simulink model "Backups"  (R2020b)
settings: Solver=VariableStepAuto  StartTime=0.0  StopTime=10.0  RelTol=1e-3
undefined symbols (not defined in the file): O, P_Blowdown, P_Needleboi
libraries: pid_lib x3, simulink x1, dspfdesign x1
(part 1 of 2)
settings Model: Creator=parthmahendru  LastModifiedBy=parthmahendru

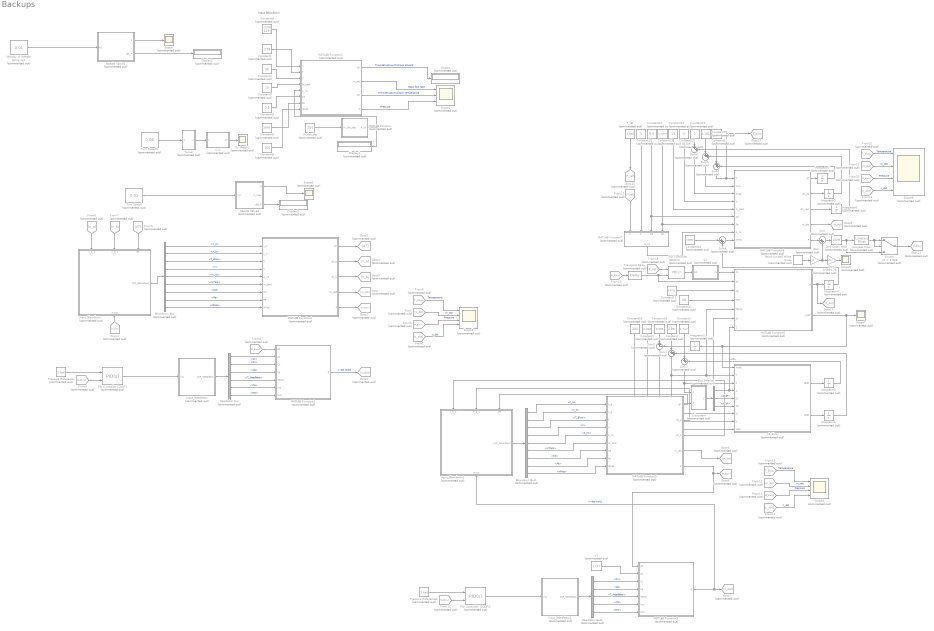
== system Backups ==
  note: Input Blowdown
  Band-Limited White Noise : simulink/Sources/Band-Limited White Noise  Commented=on  Cov=100000  Ts=0.001  seed=[23341]
  Blowdown Bus : BusSelector  Commented=on  OutputSignals=n_a,n_b,T_Blow,V,A_inj,mTank,Cd,Pe,nPres
  Blowdown Bus1 : BusSelector  Commented=on  OutputSignals=n_a,n_b,T_Blow,V,A_inj,mTank,Cd,Pe,nPres
  Bus Selector : BusSelector  Commented=on  OutputSignals=Z,dZdT,dZdP
  Constant : Constant  Commented=on  Value=298
  Constant1 : Constant  Commented=on  Value=278
  Constant10 : Constant  Commented=on
  Constant11 : Constant  Commented=on  Value=0.9723
  Constant12 : Constant  Commented=on  Value=28
  Constant13 : Constant  Commented=on  Value=10
  Constant14 : Constant  Commented=on  Value=0.0032
  Constant15 : Constant  Commented=on  Value=2.413e6  VectorParams1D=off
  Constant16 : Constant  Commented=on  Value=200
  Constant17 : Constant  Commented=on  Value=0.5
  Constant18 : Constant  Commented=on  Value=0.555
  Constant19 : Constant  Commented=on  Value=0.181
  Constant2 : Constant  Commented=on  Value=1.7e7
  Constant20 : Constant  Commented=on  Value=0.01108
  Constant21 : Constant  Commented=on  Value=0
  Constant22 : Constant  Commented=on  Value=278
  Constant3 : Constant  Commented=on  Value=30
  Constant4 : Constant  Commented=on  Value=[250 125]
  Constant5 : Constant  Commented=on  Value=10
  Constant6 : Constant  Commented=on  Value=20000
  Constant7 : Constant  Commented=on  Value=0.003
  Constant8 : Constant  Commented=on  Value=100
  Constant9 : Constant  Commented=on  Value=0.5
  Cv : Subsystem  Commented=on
  Cv Graph2 : Scope  Commented=on
  Cv1 : MATLAB Function  Commented=on  TreatAsAtomicUnit=on
  Display{,1..3} (4 alike) : Display  Commented=on
  From : From  Commented=on  GotoTag=m_dot
  From{1..2,11,16} (4 alike) : From  Commented=on  GotoTag=n_dot
  From10 : From  Commented=on  GotoTag=m_dot
  From{3..5,12..13,19..20} (7 alike) : From  Commented=on  GotoTag=P_Blow
  From14 : From  Commented=on  GotoTag=T_blow  TagVisibility=global
  From15 : From  Commented=on  GotoTag=m_dot
  From17 : From  Commented=on  GotoTag=P_ref
  From18 : From  Commented=on  GotoTag=P_ref
  From21 : From  Commented=on  GotoTag=T_blow  TagVisibility=global
  From6 : From  Commented=on  GotoTag=T_blow  TagVisibility=global
  From7 : From  Commented=on  GotoTag=n_b
  From8 : From  Commented=on  GotoTag=n_a
  From9 : From  Commented=on  GotoTag=dT
  Gain : Gain  Commented=on  Gain=4
  Gain1 : Gain  Commented=on  Gain=1/6894.76
  Goto : Goto  Commented=on  GotoTag=m_dot
  Goto1 : Goto  Commented=on  GotoTag=n_dot
  Goto10 : Goto  Commented=on  GotoTag=n_dot
  Goto11 : Goto  Commented=on  GotoTag=P_Blow
  Goto12 : Goto  Commented=on  GotoTag=T_blow  TagVisibility=global
  Goto13 : Goto  Commented=on  GotoTag=P_ref
  Goto2 : Goto  Commented=on  GotoTag=P_Blow
  Goto3 : Goto  Commented=on  GotoTag=n_b
  Goto4 : Goto  Commented=on  GotoTag=n_a
  Goto5 : Goto  Commented=on  GotoTag=dT
  Goto6 : Goto  Commented=on  GotoTag=m_dot
  Goto7 : Goto  Commented=on  GotoTag=n_dot
  Goto8 : Goto  Commented=on  GotoTag=P_Blow
  Goto9 : Goto  Commented=on  GotoTag=m_dot
  Input_Blowdown : Subsystem  Commented=on
      settings: PortSchema="{\"entries\":[{\"content\":{\"sides\":[{\"content\":{\"connectorIds\":[]},\"type\":\"ConnectorPlacement.EquallySpacedRectSide\",\"uuid\":\"6a11c464-4778-4366-9c52-25a6635196e9\"},{\"content\":{\"connectorIds\":[\"Out1\"],\"side\":\"RIGHT\"},\"type\":\"ConnectorPlacement.EquallySpacedRectSide\",\"uuid\":\"71180da6-79ed-43c5-a069-02da8079ba8e\"},{\"content\":{\"connectorIds\":[\"In1\",\"In2\",\"In3\"],\"side\":\"TOP\"},\"type\":\"ConnectorPlacement.EquallySpacedRectSide\",\"uuid\":\"0f5fbdd2-8e41-48bf-ac62-c31d274b4c94\"},{\"content\":{\"connectorIds\":[\"In4\"],\"side\":\"BOTTOM\"},\"type\":\"ConnectorPlacement.EquallySpacedRectSide\",\"uuid\":\"7608bf70-ac84-4a07-a3b2-996f245fbd8b\"}]},\"type\":\"ConnectorPlacement.EquallySpacedConnector\",\"uuid\":\"0ffd5217-2610-43b0-91a4-99377aa3c0d2\"}],\"packageUris\":[\"http://schema.mathworks.com/mf0/Connector/19700101\"],\"version\":\"1.0\"}"
  Input_Blowdown1 : Subsystem  Commented=on
      settings: PortSchema="{\"entries\":[{\"content\":{\"sides\":[{\"content\":{\"connectorIds\":[]},\"type\":\"ConnectorPlacement.EquallySpacedRectSide\",\"uuid\":\"6a11c464-4778-4366-9c52-25a6635196e9\"},{\"content\":{\"connectorIds\":[\"Out1\"],\"side\":\"RIGHT\"},\"type\":\"ConnectorPlacement.EquallySpacedRectSide\",\"uuid\":\"71180da6-79ed-43c5-a069-02da8079ba8e\"},{\"content\":{\"connectorIds\":[\"In1\",\"In2\",\"In3\"],\"side\":\"TOP\"},\"type\":\"ConnectorPlacement.EquallySpacedRectSide\",\"uuid\":\"0f5fbdd2-8e41-48bf-ac62-c31d274b4c94\"},{\"content\":{\"connectorIds\":[\"In4\"],\"side\":\"BOTTOM\"},\"type\":\"ConnectorPlacement.EquallySpacedRectSide\",\"uuid\":\"7608bf70-ac84-4a07-a3b2-996f245fbd8b\"}]},\"type\":\"ConnectorPlacement.EquallySpacedConnector\",\"uuid\":\"0ffd5217-2610-43b0-91a4-99377aa3c0d2\"}],\"packageUris\":[\"http://schema.mathworks.com/mf0/Connector/19700101\"],\"version\":\"1.0\"}"
  Input_Needleboi : Subsystem  Commented=on
  Input_Needleboi1 : Subsystem  Commented=on
  Integrator{1..7} (7 alike) : Integrator  Commented=on
  Lowpass Filter : dspfdesign/Lowpass Filter  Commented=on  FilterType=FIR  DesignForMinimumOrder=off  FilterOrder=10  PassbandFrequency=700  StopbandFrequency=3000  PassbandRipple=0.1  StopbandAttenuation=80  InheritSampleRate=off  SampleRate=44100  SimulateUsing=Interpreted execution  roundingMode=Nearest  coeffsDataTypeStr=fixdt(1,16)
  MATLAB Function : MATLAB Function  Commented=on  TreatAsAtomicUnit=on
  MATLAB Function1 : MATLAB Function  Commented=on  TreatAsAtomicUnit=on
  MATLAB Function2 : MATLAB Function  Commented=on  TreatAsAtomicUnit=on
  MATLAB Function3 : MATLAB Function  Commented=on  TreatAsAtomicUnit=on
  MATLAB Function4 : MATLAB Function  Commented=on  TreatAsAtomicUnit=on
  MATLAB Function5 : MATLAB Function  Commented=on  TreatAsAtomicUnit=on
  MATLAB Function6 : MATLAB Function  Commented=on  TreatAsAtomicUnit=on
  MATLAB Function7 : MATLAB Function  Commented=on  TreatAsAtomicUnit=on
  MATLAB Function8 : MATLAB Function  Commented=on  TreatAsAtomicUnit=on
  Needle Valve1 : Subsystem  Commented=on
  Needle Valve3 : Subsystem  Commented=on
  Needleboi Bus : BusSelector  Commented=on  OutputSignals=p1,Cv,sg,T_Needleboi,rho,MW
  Needleboi Bus1 : BusSelector  Commented=on  OutputSignals=Cv,sg,T_Needleboi,rho,MW
  PID Controller (2DOF) : pid_lib/PID Controller (2DOF)  Commented=on  Controller=PID  Form=Parallel  TimeDomain=Continuous-time  UseExternalTs=off  SampleTime=-1  IntegratorMethod=Forward Euler  FilterMethod=Forward Euler  ControllerParametersSource=internal  P=4.2846829311871e-09  I=2.39281882332403e-13  D=1.70470224737219e-05  UseFilter=on  N=1.09398371936337  b=1  c=1  TunerSelectOption=Transfer Function Based (PID Tuner App)  InitialConditionSource=internal  InitialConditionForIntegrator=0  InitialConditionForFilter=0  DifferentiatorICPrevScaledInput=0  ExternalReset=none  TrackingMode=off  Kt=1  LimitOutput=on  SatLimitsSource=internal  UpperSaturationLimit=5  LowerSaturationLimit=0  LinearizeAsGain=on  AntiWindupMode=none  Kb=1  POutMin=[]  POutMax=[]  IOutMin=[]  IOutMax=[]  DOutMin=[]  DOutMax=[]  NOutMin=[]  NOutMax=[]  bOutMin=[]  bOutMax=[]  cOutMin=[]  cOutMax=[]  SumOutMin=[]  SumOutMax=[]  SaturationOutMin=[]  SaturationOutMax=[]  PParamMin=[]  PParamMax=[]  IParamMin=[]  IParamMax=[]  DParamMin=[]  DParamMax=[]  NParamMin=[]  NParamMax=[]  bParamMin=[]  bParamMax=[]  cParamMin=[]  cParamMax=[]  KbParamMin=[]  KbParamMax=[]  KtParamMin=[]  KtParamMax=[]  KbOutMin=[]  KbOutMax=[]  KtOutMin=[]  KtOutMax=[]  IntegratorOutMin=[]  IntegratorOutMax=[]  FilterOutMin=[]  FilterOutMax=[]  SumI1OutMin=[]  SumI1OutMax=[]  SumI2OutMin=[]  SumI2OutMax=[]  SumI3OutMin=[]  SumI3OutMax=[]  SumI4OutMin=[]  SumI4OutMax=[]  SumDOutMin=[]  SumDOutMax=[]  Sum1OutMin=[]  Sum1OutMax=[]  Sum2OutMin=[]  Sum2OutMax=[]  Sum3OutMin=[]  Sum3OutMax=[]  DifferentiatorOutMin=[]  DifferentiatorOutMax=[]  FilterDiffOutCoefMin=[]  FilterDiffOutCoefMax=[]  ReciprocalOutMin=[]  ReciprocalOutMax=[]  SumDenOutMin=[]  SumDenOutMax=[]  SumNumOutMin=[]  SumNumOutMax=[]  DivideOutMin=[]  DivideOutMax=[]  UdiffTsProdOutMin=[]  UdiffTsProdOutMax=[]  NTsProdOutMin=[]  NTsProdOutMax=[]  UintegralTsProdOutMin=[]  UintegralTsProdOutMax=[]  UngainTsProdOutMin=[]  UngainTsProdOutMax=[]  IntegratorContinuousStateAttributes=''  IntegratorStateMustResolveToSignalObject=off  IntegratorRTWStateStorageClass=Auto  FilterContinuousStateAttributes=''  FilterStateMustResolveToSignalObject=off  FilterRTWStateStorageClass=Auto  ParallelPVariant=InternalParameters  IdealPVariant=Disabled  IVariant=InternalParameters  DVariant=InternalParameters  bVariant=InternalParameters  cVariant=InternalParameters  IntegratorVariant=Continuous  SatVariant=Enabled  AWVariant=Passthrough  PCopyVariant=Disabled  TRVariant=Disabled  FdbkBlocksVariant=Forward  IdealPFdbkVariant=Disabled  SatFdbkVariant=Disabled  DerivativeFilterVariant=ContFilter  NVariant=InternalParameters  NCopyVariant=Disabled  FilterICVariant=InternalICsFilter  IntegratorICVariant=InternalICs  ExternalResetVariant=Disabled  TRSumVariant=Passthrough  SumFdbkVariant=Disabled  SumVariant=Sum_PID  TsampFilterVariant=InternalTs  TsampNgainVariant=Passthrough  TsampIntegralVariant=Passthrough  ExternalSaturationOutDataTypeStr=Inherit: Same as second input
      settings: SourceProductBaseCode=SL
  PID Controller (2DOF)1 : pid_lib/PID Controller (2DOF)  Commented=on  Controller=PID  Form=Parallel  TimeDomain=Continuous-time  UseExternalTs=off  SampleTime=-1  IntegratorMethod=Forward Euler  FilterMethod=Forward Euler  ControllerParametersSource=internal  P=4.2846829311871e-09  I=2.39281882332403e-13  D=1.70470224737219e-05  UseFilter=on  N=1.09398371936337  b=1  c=1  TunerSelectOption=Transfer Function Based (PID Tuner App)  InitialConditionSource=internal  InitialConditionForIntegrator=0  InitialConditionForFilter=0  DifferentiatorICPrevScaledInput=0  ExternalReset=none  TrackingMode=off  Kt=1  LimitOutput=on  SatLimitsSource=internal  UpperSaturationLimit=5  LowerSaturationLimit=0  LinearizeAsGain=on  AntiWindupMode=none  Kb=1  POutMin=[]  POutMax=[]  IOutMin=[]  IOutMax=[]  DOutMin=[]  DOutMax=[]  NOutMin=[]  NOutMax=[]  bOutMin=[]  bOutMax=[]  cOutMin=[]  cOutMax=[]  SumOutMin=[]  SumOutMax=[]  SaturationOutMin=[]  SaturationOutMax=[]  PParamMin=[]  PParamMax=[]  IParamMin=[]  IParamMax=[]  DParamMin=[]  DParamMax=[]  NParamMin=[]  NParamMax=[]  bParamMin=[]  bParamMax=[]  cParamMin=[]  cParamMax=[]  KbParamMin=[]  KbParamMax=[]  KtParamMin=[]  KtParamMax=[]  KbOutMin=[]  KbOutMax=[]  KtOutMin=[]  KtOutMax=[]  IntegratorOutMin=[]  IntegratorOutMax=[]  FilterOutMin=[]  FilterOutMax=[]  SumI1OutMin=[]  SumI1OutMax=[]  SumI2OutMin=[]  SumI2OutMax=[]  SumI3OutMin=[]  SumI3OutMax=[]  SumI4OutMin=[]  SumI4OutMax=[]  SumDOutMin=[]  SumDOutMax=[]  Sum1OutMin=[]  Sum1OutMax=[]  Sum2OutMin=[]  Sum2OutMax=[]  Sum3OutMin=[]  Sum3OutMax=[]  DifferentiatorOutMin=[]  DifferentiatorOutMax=[]  FilterDiffOutCoefMin=[]  FilterDiffOutCoefMax=[]  ReciprocalOutMin=[]  ReciprocalOutMax=[]  SumDenOutMin=[]  SumDenOutMax=[]  SumNumOutMin=[]  SumNumOutMax=[]  DivideOutMin=[]  DivideOutMax=[]  UdiffTsProdOutMin=[]  UdiffTsProdOutMax=[]  NTsProdOutMin=[]  NTsProdOutMax=[]  UintegralTsProdOutMin=[]  UintegralTsProdOutMax=[]  UngainTsProdOutMin=[]  UngainTsProdOutMax=[]  IntegratorContinuousStateAttributes=''  IntegratorStateMustResolveToSignalObject=off  IntegratorRTWStateStorageClass=Auto  FilterContinuousStateAttributes=''  FilterStateMustResolveToSignalObject=off  FilterRTWStateStorageClass=Auto  ParallelPVariant=InternalParameters  IdealPVariant=Disabled  IVariant=InternalParameters  DVariant=InternalParameters  bVariant=InternalParameters  cVariant=InternalParameters  IntegratorVariant=Continuous  SatVariant=Enabled  AWVariant=Passthrough  PCopyVariant=Disabled  TRVariant=Disabled  FdbkBlocksVariant=Forward  IdealPFdbkVariant=Disabled  SatFdbkVariant=Disabled  DerivativeFilterVariant=ContFilter  NVariant=InternalParameters  NCopyVariant=Disabled  FilterICVariant=InternalICsFilter  IntegratorICVariant=InternalICs  ExternalResetVariant=Disabled  TRSumVariant=Passthrough  SumFdbkVariant=Disabled  SumVariant=Sum_PID  TsampFilterVariant=InternalTs  TsampNgainVariant=Passthrough  TsampIntegralVariant=Passthrough  ExternalSaturationOutDataTypeStr=Inherit: Same as second input
      settings: SourceProductBaseCode=SL
  PID Controller (2DOF)2 : pid_lib/PID Controller (2DOF)  Commented=on  Controller=PD  Form=Parallel  TimeDomain=Continuous-time  UseExternalTs=off  SampleTime=-1  IntegratorMethod=Forward Euler  FilterMethod=Forward Euler  ControllerParametersSource=internal  P=3.2e-09  I=1.39281882332403e-13  D=0.9e-05  UseFilter=on  N=1.09398371936337  b=1  c=1  TunerSelectOption=Transfer Function Based (PID Tuner App)  InitialConditionSource=internal  InitialConditionForIntegrator=0  InitialConditionForFilter=0  DifferentiatorICPrevScaledInput=0  ExternalReset=none  TrackingMode=off  Kt=1  LimitOutput=on  SatLimitsSource=internal  UpperSaturationLimit=5  LowerSaturationLimit=0  LinearizeAsGain=on  AntiWindupMode=none  Kb=1  POutMin=[]  POutMax=[]  IOutMin=[]  IOutMax=[]  DOutMin=[]  DOutMax=[]  NOutMin=[]  NOutMax=[]  bOutMin=[]  bOutMax=[]  cOutMin=[]  cOutMax=[]  SumOutMin=[]  SumOutMax=[]  SaturationOutMin=[]  SaturationOutMax=[]  PParamMin=[]  PParamMax=[]  IParamMin=[]  IParamMax=[]  DParamMin=[]  DParamMax=[]  NParamMin=[]  NParamMax=[]  bParamMin=[]  bParamMax=[]  cParamMin=[]  cParamMax=[]  KbParamMin=[]  KbParamMax=[]  KtParamMin=[]  KtParamMax=[]  KbOutMin=[]  KbOutMax=[]  KtOutMin=[]  KtOutMax=[]  IntegratorOutMin=[]  IntegratorOutMax=[]  FilterOutMin=[]  FilterOutMax=[]  SumI1OutMin=[]  SumI1OutMax=[]  SumI2OutMin=[]  SumI2OutMax=[]  SumI3OutMin=[]  SumI3OutMax=[]  SumI4OutMin=[]  SumI4OutMax=[]  SumDOutMin=[]  SumDOutMax=[]  Sum1OutMin=[]  Sum1OutMax=[]  Sum2OutMin=[]  Sum2OutMax=[]  Sum3OutMin=[]  Sum3OutMax=[]  DifferentiatorOutMin=[]  DifferentiatorOutMax=[]  FilterDiffOutCoefMin=[]  FilterDiffOutCoefMax=[]  ReciprocalOutMin=[]  ReciprocalOutMax=[]  SumDenOutMin=[]  SumDenOutMax=[]  SumNumOutMin=[]  SumNumOutMax=[]  DivideOutMin=[]  DivideOutMax=[]  UdiffTsProdOutMin=[]  UdiffTsProdOutMax=[]  NTsProdOutMin=[]  NTsProdOutMax=[]  UintegralTsProdOutMin=[]  UintegralTsProdOutMax=[]  UngainTsProdOutMin=[]  UngainTsProdOutMax=[]  IntegratorContinuousStateAttributes=''  IntegratorStateMustResolveToSignalObject=off  IntegratorRTWStateStorageClass=Auto  FilterContinuousStateAttributes=''  FilterStateMustResolveToSignalObject=off  FilterRTWStateStorageClass=Auto  ParallelPVariant=InternalParameters  IdealPVariant=Disabled  IVariant=Disabled  DVariant=InternalParameters  bVariant=InternalParameters  cVariant=InternalParameters  IntegratorVariant=Disabled  SatVariant=Enabled  AWVariant=Disabled  PCopyVariant=Disabled  TRVariant=Disabled  FdbkBlocksVariant=Forward  IdealPFdbkVariant=Disabled  SatFdbkVariant=Disabled  DerivativeFilterVariant=ContFilter  NVariant=InternalParameters  NCopyVariant=Disabled  FilterICVariant=InternalICsFilter  IntegratorICVariant=Disabled  ExternalResetVariant=Disabled  TRSumVariant=Passthrough  SumFdbkVariant=Disabled  SumVariant=Sum_PD  TsampFilterVariant=InternalTs  TsampNgainVariant=Passthrough  TsampIntegralVariant=Disabled_SignalSpec  ExternalSaturationOutDataTypeStr=Inherit: Same as second input
      settings: SourceProductBaseCode=SL
  P_ref : Constant  Commented=on  Value=3.6e6
  Pressure Reference : Constant  Commented=on  Value=3.6e6
  Pressure Reference1 : Constant  Commented=on  Value=3.6e6
  Scope{,2,5,7} (4 alike) : Scope  Commented=on
  Scope1 : Scope  Commented=on  NumInputPorts=3
  Scope3 : Scope  Commented=on  NumInputPorts=4
  Scope4 : Scope  Commented=on  NumInputPorts=4
  Scope6 : Scope  Commented=on  NumInputPorts=4
  Subsystem : Subsystem  Commented=on
  Sum{,1..2,4..7} (7 alike) : Sum  Commented=on  Inputs=|++
  Sum3 : Sum  Commented=on  Inputs=|+-
  Switch : Switch  Commented=on  Criteria=u2 > Threshold  Threshold=3.5e6
  Transport Delay : TransportDelay  Commented=on  DelayTime=0.01
  Turn Speed : Constant  Commented=on  Value=0.01  VectorParams1D=off
  Turn Speed2 : Constant  Commented=on  Value=0.08  VectorParams1D=off
  Turner : Subsystem  Commented=on
  Velocity of Needle going up1 : Constant  Commented=on  Value=0.01  VectorParams1D=off
  Zero-Order Hold : ZeroOrderHold  Commented=on  SampleTime=-1
  m_dot_des : Constant  Commented=on  Value=250
  n2_blow : MATLAB Function  Commented=on  TreatAsAtomicUnit=on
  p1 : Constant  Commented=on  Value=1.7e7
  wires:
  Constant8/1 -> MATLAB Function2/8(nPres)
  MATLAB Function2/2(m_dot) -> Scope1/1  "Mass flow rate"
  Constant3/1 -> MATLAB Function2/3(V)
  Needle Valve1/2(del_P) -> Display2/1
  MATLAB Function/1(A_inj) -> Display1/1, MATLAB Function2/5(A_inj)
  Velocity of Needle going up1/1 -> Needle Valve1/1(In1)
  Constant5/1 -> MATLAB Function2/4(m_tank)
  Needle Valve1/1(q) -> Scope/1
  MATLAB Function2/3(dT) -> Scope1/2  "Time derivative of tank temperature"
  Constant4/1 -> MATLAB Function2/1(n)
  MATLAB Function2/4(P) -> Scope1/3  "Pressure"
  MATLAB Function2/1(dn) -> Display/1  "Time derivative of nitrous amount"
  Constant1/1 -> MATLAB Function2/2(T)
  Constant9/1 -> MATLAB Function2/6(Cd)
  m_dot_des/1 -> MATLAB Function/1(m_dot_des)
  Constant6/1 -> MATLAB Function2/7(Pe)
  Turn Speed/1 -> Needle Valve3/1(In1)
  Needle Valve3/1(q) -> Scope2/1
  Turn Speed2/1 -> Turner/1(In1)
  Needle Valve3/3(del_P) -> Display3/1
  Cv1/1(Cv) -> Cv Graph2/1
  Turner/1(Out1) -> Cv1/1(u)
  Pressure Reference/1 -> PID Controller (2DOF)/1
  Blowdown Bus/7 -> MATLAB Function4/7(Cd)  "<Cd>"
  Blowdown Bus/3 -> MATLAB Function4/3(T)  "<T_Blow>"
  Blowdown Bus/2 -> MATLAB Function4/2(n_b)  "<n_b>"
  From/1 -> Scope3/2  "m_dot"
  From8/1 -> Input_Blowdown/1(n_a_1)
  Blowdown Bus/4 -> MATLAB Function4/4(V)  "<V>"
  Blowdown Bus/8 -> MATLAB Function4/8(Pe)  "<Pe>"
  Blowdown Bus/9 -> MATLAB Function4/9(nPres)  "<nPres>"
  Blowdown Bus/6 -> MATLAB Function4/6(m_tank)  "<mTank>"
  MATLAB Function1/1(q) -> Goto1/1  "n -dot mol/s"
  From7/1 -> Input_Blowdown/2(n_b_1)
  Needleboi Bus/5 -> MATLAB Function1/6(rho)  "<rho>"
  Needleboi Bus/2 -> MATLAB Function1/3(Cv)  "<Cv>"
  From9/1 -> Input_Blowdown/3(dT)
  MATLAB Function4/2(dn_a) -> Goto4/1
  Needleboi Bus/3 -> MATLAB Function1/4(sg)  "<sg>"
  Needleboi Bus/6 -> MATLAB Function1/7(MW)  "<MW>"
  From6/1 -> Scope3/1  "Temperature"
  MATLAB Function4/3(dn_b) -> Goto3/1
  MATLAB Function4/5(P) -> Goto2/1
  Needleboi Bus/1 -> MATLAB Function1/2(p1)  "<p1>"
  Input_Needleboi/1(O/P_Needleboi) -> Needleboi Bus/1
  Needleboi Bus/4 -> MATLAB Function1/5(Temp)  "<T_Needleboi>"
  Blowdown Bus/5 -> MATLAB Function4/5(A_inj)  "<A_inj>"
  PID Controller (2DOF)/1 -> Input_Needleboi/1(In1)
  From1/1 -> Scope3/4  "n_dot"
  Input_Blowdown/1(O/P_Blowdown) -> Blowdown Bus/1
  Blowdown Bus/1 -> MATLAB Function4/1(n_a)  "<n_a>"
  From3/1 -> PID Controller (2DOF)/2
  From4/1 -> MATLAB Function1/1(p2)
  From5/1 -> Scope3/3  "Pressure"
  From2/1 -> Input_Blowdown/4(mol/s)
  MATLAB Function4/4(m_dot) -> Goto/1
  MATLAB Function4/1(dT) -> Goto5/1
  Blowdown Bus1/4 -> MATLAB Function5/4(V)  "<V>"
  Pressure Reference1/1 -> PID Controller (2DOF)1/1
  Blowdown Bus1/2 -> MATLAB Function5/2(n_b)  "<n_b>"
  MATLAB Function5/5(P) -> MATLAB Function3/1(p2), Goto8/1
  Needleboi Bus1/1 -> MATLAB Function3/3(Cv)  "<Cv>"
  Needleboi Bus1/4 -> MATLAB Function3/6(rho)  "<rho>"
  MATLAB Function3/1(q) -> Goto7/1, Input_Blowdown1/4(mol/s)  "n -dot mol/s"
  Blowdown Bus1/9 -> MATLAB Function5/9(nPres)  "<nPres>"
  Blowdown Bus1/6 -> MATLAB Function5/6(m_tank)  "<mTank>"
  Blowdown Bus1/7 -> MATLAB Function5/7(Cd)  "<Cd>"
  PID Controller (2DOF)1/1 -> Input_Needleboi1/1(In1)
  Blowdown Bus1/1 -> MATLAB Function5/1(n_a)  "<n_a>"
  Needleboi Bus1/3 -> MATLAB Function3/5(Temp)  "<T_Needleboi>"
  Needleboi Bus1/5 -> MATLAB Function3/7(MW)  "<MW>"
  MATLAB Function5/3(dn_b) -> Input_Blowdown1/1(n_b_1)
  Input_Blowdown1/1(O/P_Blowdown) -> Blowdown Bus1/1
  Needleboi Bus1/2 -> MATLAB Function3/4(sg)  "<sg>"
  Blowdown Bus1/8 -> MATLAB Function5/8(Pe)  "<Pe>"
  MATLAB Function5/4(m_dot) -> Goto6/1
  MATLAB Function5/1(dT) -> Input_Blowdown1/3(dT)
  Input_Needleboi1/1(O/P_Needleboi) -> Needleboi Bus1/1
  From12/1 -> PID Controller (2DOF)1/2
  From14/1 -> Scope4/1  "Temperature"
  From10/1 -> Scope4/2  "m_dot"
  Blowdown Bus1/3 -> MATLAB Function5/3(T)  "<T_Blow>"
  Blowdown Bus1/5 -> MATLAB Function5/5(A_inj)  "<A_inj>"
  From11/1 -> Scope4/4  "n_dot"
  From13/1 -> Scope4/3  "Pressure"
  MATLAB Function5/2(dn_a) -> Input_Blowdown1/2(n_a_1)
  p1/1 -> MATLAB Function3/2(p1)
  Transport Delay/1 -> MATLAB Function6/2(p2), PID Controller (2DOF)2/2
  n2_blow/1(dPdt) -> Integrator2/1
  MATLAB Function8/4(m_dot) -> Goto9/1
  n2_blow/2(dTdt) -> Integrator1/1
  P_ref/1 -> Goto13/1
  Sum2/1 -> MATLAB Function6/6(p1), n2_blow/3(P), Subsystem/1(P)
  Subsystem/1(Outport) -> Bus Selector/1
  MATLAB Function8/5(P) -> Sum/1
  From19/1 -> Transport Delay/1
  Gain/1 -> Sum/2, Gain1/1
  From17/1 -> MATLAB Function7/1(P)
  Constant10/1 -> MATLAB Function7/2(m_dot_des)
  Integrator1/1 -> Sum1/2
  From18/1 -> PID Controller (2DOF)2/1
  Sum7/1 -> Goto12/1, MATLAB Function8/1(T)
  Sum1/1 -> MATLAB Function6/5(Temp), n2_blow/2(T), Subsystem/2(T)
  Constant15/1 -> MATLAB Function7/4(Pe), MATLAB Function8/7(Pe)
  Bus Selector/2 -> n2_blow/5(Zt)  "<dZdT>"
  Sum4/1 -> MATLAB Function8/9(nPres)
  From20/1 -> Scope6/3  "Pressure"
  Lowpass Filter/1 -> Switch/2, Switch/1
  Integrator7/1 -> Sum7/2
  Constant19/1 -> Sum5/1
  From16/1 -> Scope6/4  "n_dot"
  Bus Selector/3 -> n2_blow/6(Zb)  "<dZdP>"
  Constant21/1 -> Sum6/1
  Bus Selector/1 -> MATLAB Function6/7(Z), n2_blow/4(Z)  "<Z>"
  MATLAB Function6/1(q) -> Goto10/1, Integrator4/1
  Sum3/1 -> n2_blow/7(m)
  Integrator5/1 -> Sum5/2
  Switch/1 -> Goto11/1
  Constant11/1 -> MATLAB Function6/3(sg)
  Sum5/1 -> MATLAB Function8/2(nLiq)
  Zero-Order Hold/1 -> Lowpass Filter/1, Switch/3
  Constant12/1 -> MATLAB Function6/4(MW)
  PID Controller (2DOF)2/1 -> Cv/1(In1)
  Band-Limited White Noise/1 -> Gain/1
  From15/1 -> Scope6/2  "m_dot"
  Constant16/1 -> n2_blow/9(qdot)
  Constant7/1 -> n2_blow/8(V)
  Constant2/1 -> Sum2/1
  Constant18/1 -> Sum3/1
  Constant17/1 -> MATLAB Function7/3(Cd), MATLAB Function8/6(Cd)
  MATLAB Function7/1(A_inj) -> MATLAB Function8/8(A_inj)
  MATLAB Function6/2(mdot) -> Scope7/1, n2_blow/1(mdot), Integrator3/1
  Integrator3/1 -> Sum3/2
  Constant20/1 -> MATLAB Function8/4(V)
  MATLAB Function8/2(dn_liq) -> Integrator5/1
  Sum6/1 -> MATLAB Function8/3(nVap)
  Constant/1 -> Sum1/1
  Constant22/1 -> Sum7/1
  MATLAB Function8/3(dn_vap) -> Integrator6/1
  MATLAB Function8/1(dT) -> Integrator7/1
  Integrator4/1 -> Sum4/2
  Constant13/1 -> MATLAB Function8/5(m_tank)
  Integrator2/1 -> Sum2/2
  Constant14/1 -> Sum4/1
  From21/1 -> Scope6/1  "Temperature"
  Gain1/1 -> Scope5/1
  Sum/1 -> Zero-Order Hold/1
  Integrator6/1 -> Sum6/2
  Cv/1(cv) -> MATLAB Function6/1(Cv)

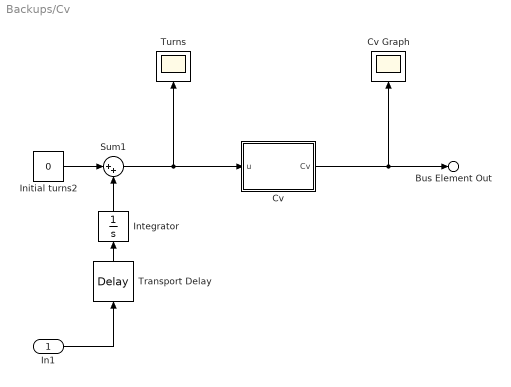
== system Backups/Cv ==
  In1 : Inport
  Cv : MATLAB Function  TreatAsAtomicUnit=on
  Cv Graph : Scope
  Initial turns2 : Constant  Value=0
  Integrator : Integrator
  Sum1 : Sum  Inputs=|++
  Transport Delay : TransportDelay  DelayTime=0.004
  Turns : Scope
  Bus Element Out : Outport  PortName=cv  Element=signal1
  wires:
  In1/1 -> Transport Delay/1
  Integrator/1 -> Sum1/2
  Initial turns2/1 -> Sum1/1
  Cv/1(Cv) -> Cv Graph/1, Bus Element Out/1
  Sum1/1 -> Cv/1(u), Turns/1
  Transport Delay/1 -> Integrator/1

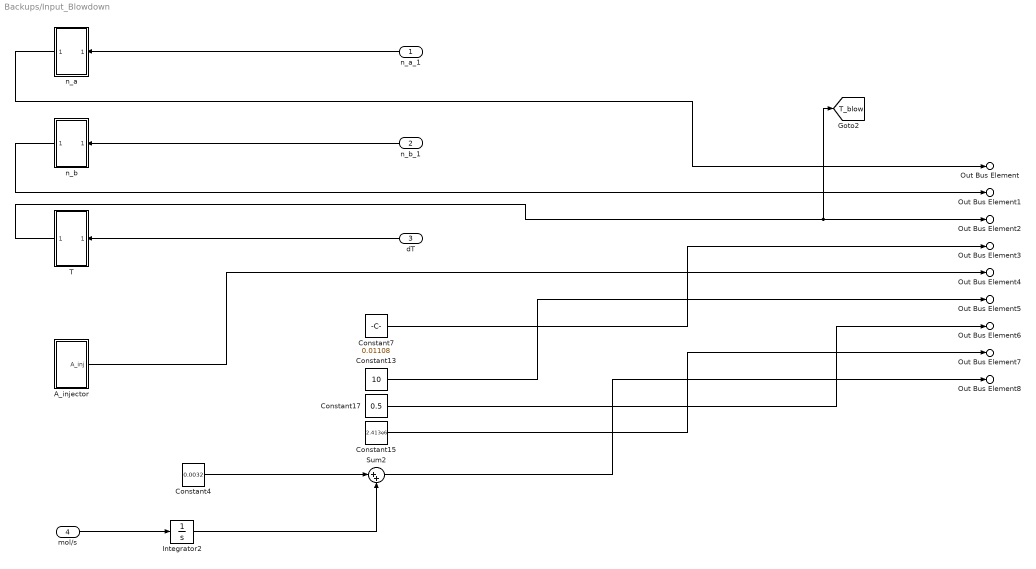
== system Backups/Input_Blowdown ==
  n_a_1 : Inport
  n_b_1 : Inport  Port=2
  dT : Inport  Port=3
  mol/s : Inport  Port=4
  A_injector : Subsystem
  Constant13 : Constant  Value=10
  Constant15 : Constant  Value=2.413e6  VectorParams1D=off
  Constant17 : Constant  Value=0.5
  Constant4 : Constant  Value=0.0032
  Constant7 : Constant  Value=0.01108
  Integrator2 : Integrator
  Sum2 : Sum  Inputs=|++
  T : Subsystem
  n_a : Subsystem
  n_b : Subsystem
  Out Bus Element : Outport  PortName=O/P_Blowdown  Element=n_a
  Out Bus Element1 : Outport  PortName=O/P_Blowdown  Element=n_b
  Out Bus Element2 : Outport  PortName=O/P_Blowdown  Element=T_Blow
  Out Bus Element3 : Outport  PortName=O/P_Blowdown  Element=V
  Out Bus Element4 : Outport  PortName=O/P_Blowdown  Element=A_inj
  Out Bus Element5 : Outport  PortName=O/P_Blowdown  Element=mTank
  Out Bus Element6 : Outport  PortName=O/P_Blowdown  Element=Cd
  Out Bus Element7 : Outport  PortName=O/P_Blowdown  Element=Pe
  Out Bus Element8 : Outport  PortName=O/P_Blowdown  Element=nPres
  tag scope: T_blow=global
  wires:
  A_injector/1(A_inj) -> Out Bus Element4/1
  T/1(Out1) -> [T_blow], Out Bus Element2/1
  n_a/1(O/P_Blowdown) -> Out Bus Element/1
  mol/s/1 -> Integrator2/1
  Constant7/1 -> Out Bus Element3/1
  Sum2/1 -> Out Bus Element8/1
  Constant4/1 -> Sum2/1
  Constant13/1 -> Out Bus Element5/1
  Constant15/1 -> Out Bus Element7/1
  n_b/1(n_b) -> Out Bus Element1/1
  Constant17/1 -> Out Bus Element6/1
  n_a_1/1 -> n_a/1(In1)
  dT/1 -> T/1(Time derivative)
  n_b_1/1 -> n_b/1(In1)
  Integrator2/1 -> Sum2/2

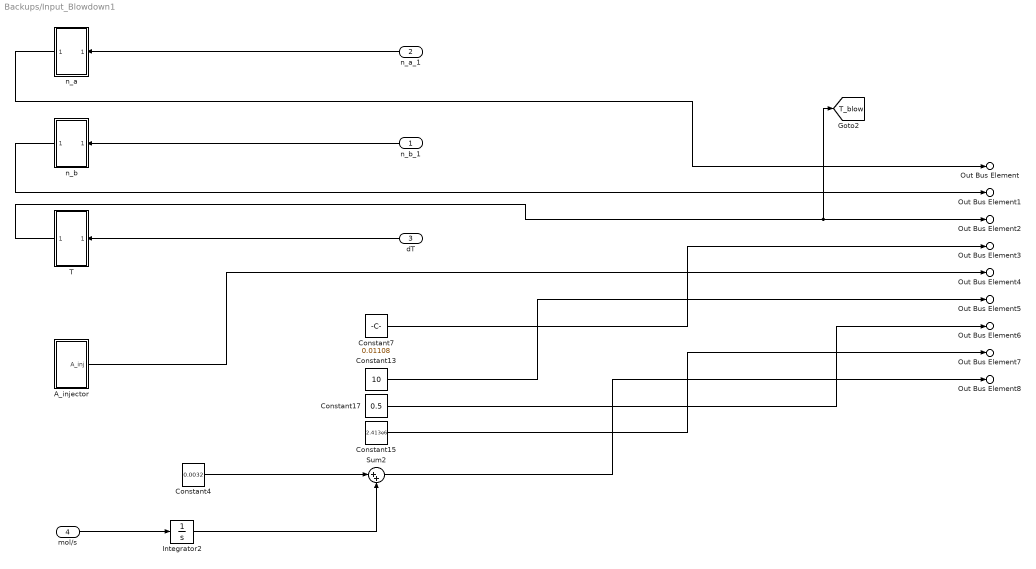
== system Backups/Input_Blowdown1 ==
  n_b_1 : Inport
  n_a_1 : Inport  Port=2
  dT : Inport  Port=3
  mol/s : Inport  Port=4
  A_injector : Subsystem
  Constant13 : Constant  Value=10
  Constant15 : Constant  Value=2.413e6  VectorParams1D=off
  Constant17 : Constant  Value=0.5
  Constant4 : Constant  Value=0.0032
  Constant7 : Constant  Value=0.01108
  Integrator2 : Integrator
  Sum2 : Sum  Inputs=|++
  T : Subsystem
  n_a : Subsystem
  n_b : Subsystem
  Out Bus Element : Outport  PortName=O/P_Blowdown  Element=n_a
  Out Bus Element1 : Outport  PortName=O/P_Blowdown  Element=n_b
  Out Bus Element2 : Outport  PortName=O/P_Blowdown  Element=T_Blow
  Out Bus Element3 : Outport  PortName=O/P_Blowdown  Element=V
  Out Bus Element4 : Outport  PortName=O/P_Blowdown  Element=A_inj
  Out Bus Element5 : Outport  PortName=O/P_Blowdown  Element=mTank
  Out Bus Element6 : Outport  PortName=O/P_Blowdown  Element=Cd
  Out Bus Element7 : Outport  PortName=O/P_Blowdown  Element=Pe
  Out Bus Element8 : Outport  PortName=O/P_Blowdown  Element=nPres
  tag scope: T_blow=global
  wires:
  A_injector/1(A_inj) -> Out Bus Element4/1
  T/1(Out1) -> [T_blow], Out Bus Element2/1
  n_a/1(O/P_Blowdown) -> Out Bus Element/1
  mol/s/1 -> Integrator2/1
  Constant7/1 -> Out Bus Element3/1
  Sum2/1 -> Out Bus Element8/1
  Constant4/1 -> Sum2/1
  Constant13/1 -> Out Bus Element5/1
  Constant15/1 -> Out Bus Element7/1
  n_b/1(n_b) -> Out Bus Element1/1
  Constant17/1 -> Out Bus Element6/1
  n_a_1/1 -> n_a/1(In1)
  dT/1 -> T/1(Time derivative)
  n_b_1/1 -> n_b/1(In1)
  Integrator2/1 -> Sum2/2

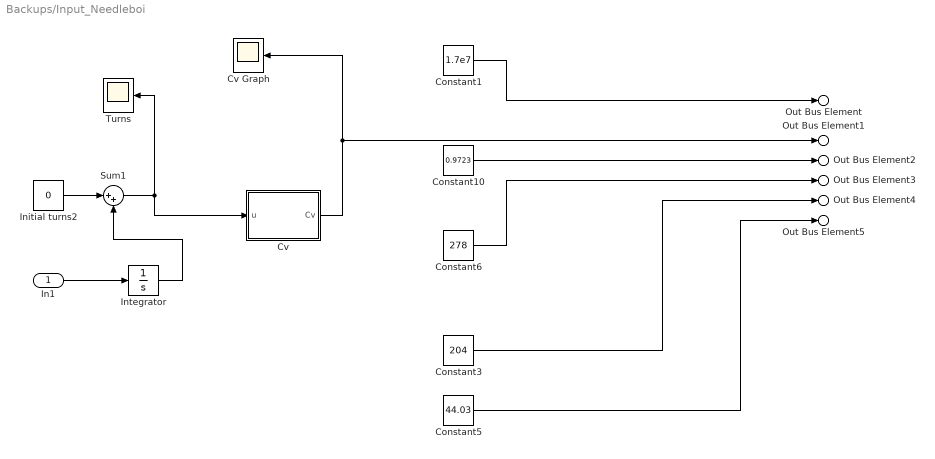
== system Backups/Input_Needleboi ==
  In1 : Inport
  Constant1 : Constant  Value=1.7e7
  Constant10 : Constant  Value=0.9723
  Constant3 : Constant  Value=204
  Constant5 : Constant  Value=44.03
  Constant6 : Constant  Value=278
  Cv : MATLAB Function  TreatAsAtomicUnit=on
  Cv Graph : Scope
  Initial turns2 : Constant  Value=0
  Integrator : Integrator
  Sum1 : Sum  Inputs=|++
  Turns : Scope
  Out Bus Element : Outport  PortName=O/P_Needleboi  Element=p1
  Out Bus Element1 : Outport  PortName=O/P_Needleboi  Element=Cv
  Out Bus Element2 : Outport  PortName=O/P_Needleboi  Element=sg
  Out Bus Element3 : Outport  PortName=O/P_Needleboi  Element=T_Needleboi
  Out Bus Element4 : Outport  PortName=O/P_Needleboi  Element=rho
  Out Bus Element5 : Outport  PortName=O/P_Needleboi  Element=MW
  wires:
  In1/1 -> Integrator/1
  Constant3/1 -> Out Bus Element4/1
  Constant1/1 -> Out Bus Element/1
  Constant5/1 -> Out Bus Element5/1
  Integrator/1 -> Sum1/2
  Constant10/1 -> Out Bus Element2/1
  Initial turns2/1 -> Sum1/1
  Cv/1(Cv) -> Out Bus Element1/1, Cv Graph/1
  Constant6/1 -> Out Bus Element3/1
  Sum1/1 -> Turns/1, Cv/1(u)

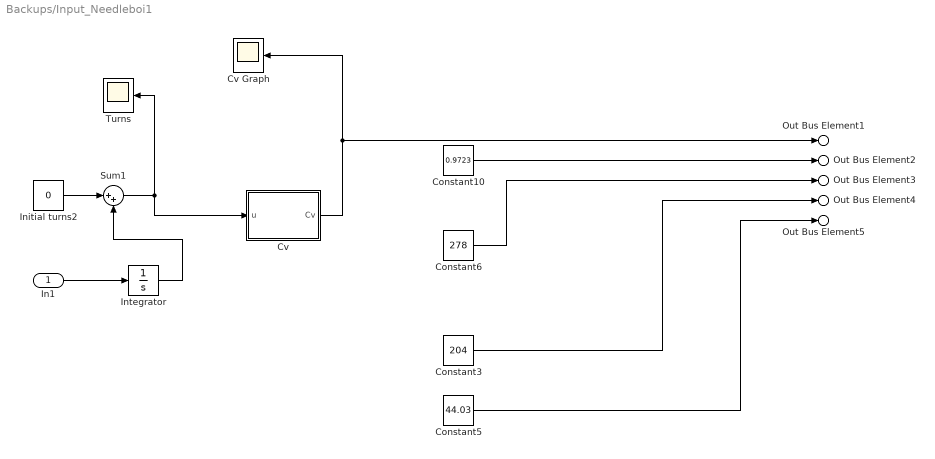
== system Backups/Input_Needleboi1 ==
  In1 : Inport
  Constant10 : Constant  Value=0.9723
  Constant3 : Constant  Value=204
  Constant5 : Constant  Value=44.03
  Constant6 : Constant  Value=278
  Cv : MATLAB Function  TreatAsAtomicUnit=on
  Cv Graph : Scope
  Initial turns2 : Constant  Value=0
  Integrator : Integrator
  Sum1 : Sum  Inputs=|++
  Turns : Scope
  Out Bus Element1 : Outport  PortName=O/P_Needleboi  Element=Cv
  Out Bus Element2 : Outport  PortName=O/P_Needleboi  Element=sg
  Out Bus Element3 : Outport  PortName=O/P_Needleboi  Element=T_Needleboi
  Out Bus Element4 : Outport  PortName=O/P_Needleboi  Element=rho
  Out Bus Element5 : Outport  PortName=O/P_Needleboi  Element=MW
  wires:
  In1/1 -> Integrator/1
  Constant3/1 -> Out Bus Element4/1
  Constant5/1 -> Out Bus Element5/1
  Integrator/1 -> Sum1/2
  Constant10/1 -> Out Bus Element2/1
  Initial turns2/1 -> Sum1/1
  Cv/1(Cv) -> Out Bus Element1/1, Cv Graph/1
  Constant6/1 -> Out Bus Element3/1
  Sum1/1 -> Turns/1, Cv/1(u)

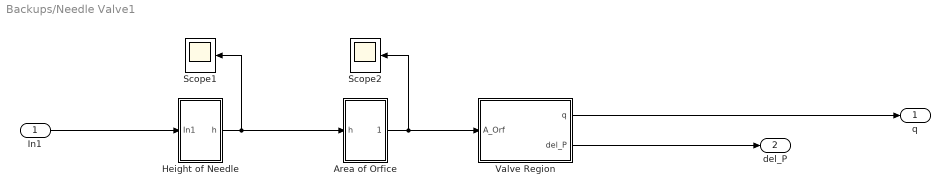
== system Backups/Needle Valve1 ==
  In1 : Inport
  Area of Orfice : Subsystem
  Height of Needle : Subsystem
  Scope1 : Scope
  Scope2 : Scope
  Valve Region : Subsystem
  q : Outport
  del_P : Outport  Port=2
  wires:
  Valve Region/2(del_P) -> del_P/1
  Valve Region/1(q) -> q/1
  Height of Needle/1(h) -> Area of Orfice/1(h), Scope1/1
  In1/1 -> Height of Needle/1(In1)
  Area of Orfice/1(A_Orf) -> Valve Region/1(A_Orf), Scope2/1

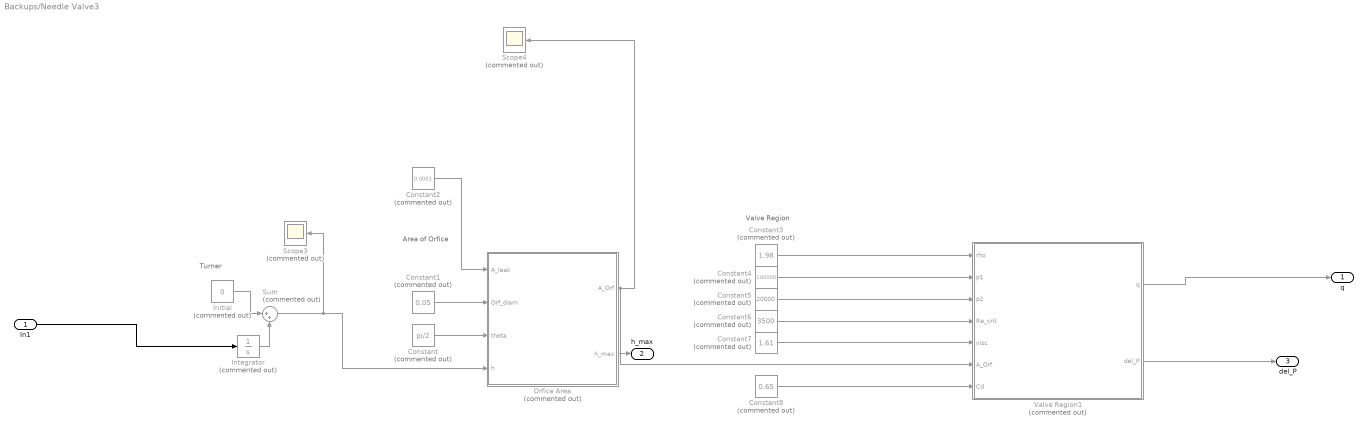
== system Backups/Needle Valve3 ==
  note: Valve Region
  note: Area of Orfice
  note: Turner
  In1 : Inport
  Constant : Constant  Commented=on  Value=pi/2
  Constant1 : Constant  Commented=on  Value=0.05
  Constant2 : Constant  Commented=on  Value=0.0001
  Constant3 : Constant  Commented=on  Value=1.98
  Constant4 : Constant  Commented=on  Value=100000
  Constant5 : Constant  Commented=on  Value=20000
  Constant6 : Constant  Commented=on  Value=3500
  Constant7 : Constant  Commented=on  Value=1.61
  Constant8 : Constant  Commented=on  Value=0.65
  "Initial " : Constant  Commented=on  Value=0
  Integrator : Integrator  Commented=on
  Orfice Area : MATLAB Function  Commented=on  TreatAsAtomicUnit=on
  Scope3 : Scope  Commented=on
  Scope4 : Scope  Commented=on
  Sum : Sum  Commented=on  Inputs=|++
  Valve Region1 : MATLAB Function  Commented=on  TreatAsAtomicUnit=on
  q : Outport
  h_max : Outport  Port=2
  del_P : Outport  Port=3
  wires:
  Valve Region1/2(del_P) -> del_P/1
  Constant1/1 -> Orfice Area/2(Orf_diam)
  "Initial "/1 -> Sum/1
  Constant6/1 -> Valve Region1/4(Re_crit)
  Constant3/1 -> Valve Region1/1(rho)
  Constant5/1 -> Valve Region1/3(p2)
  In1/1 -> Integrator/1
  Valve Region1/1(q) -> q/1
  Sum/1 -> Scope3/1, Orfice Area/4(h)
  Constant2/1 -> Orfice Area/1(A_leak)
  Constant7/1 -> Valve Region1/5(visc)
  Orfice Area/1(A_Orf) -> Valve Region1/6(A_Orf), Scope4/1
  Constant4/1 -> Valve Region1/2(p1)
  Orfice Area/2(h_max) -> h_max/1
  Integrator/1 -> Sum/2
  Constant/1 -> Orfice Area/3(theta)
  Constant8/1 -> Valve Region1/7(Cd)

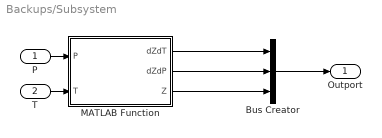
== system Backups/Subsystem ==
  P : Inport
  T : Inport  Port=2
  Bus Creator : BusCreator  Inputs=3
  MATLAB Function : MATLAB Function  TreatAsAtomicUnit=on
  Outport : Outport
  wires:
  MATLAB Function/1(dZdT) -> Bus Creator/1
  T/1 -> MATLAB Function/2(T)
  MATLAB Function/2(dZdP) -> Bus Creator/2
  P/1 -> MATLAB Function/1(P)
  MATLAB Function/3(Z) -> Bus Creator/3
  Bus Creator/1 -> Outport/1

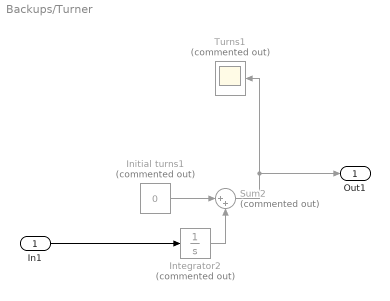
== system Backups/Turner ==
  In1 : Inport
  Initial turns1 : Constant  Commented=on  Value=0
  Integrator2 : Integrator  Commented=on
  Sum2 : Sum  Commented=on  Inputs=|++
  Turns1 : Scope  Commented=on
  Out1 : Outport
  wires:
  Initial turns1/1 -> Sum2/1
  In1/1 -> Integrator2/1
  Integrator2/1 -> Sum2/2
  Sum2/1 -> Out1/1, Turns1/1

== system Backups/Input_Blowdown/A_injector ==
  Display1 : Display
  MATLAB Function1 : MATLAB Function  TreatAsAtomicUnit=on
  m_dot_des2 : Constant
  A_inj : Outport
  wires:
  MATLAB Function1/1(A_inj) -> A_inj/1, Display1/1
  m_dot_des2/1 -> MATLAB Function1/1(m_dot_des)

== system Backups/Input_Blowdown/T ==
  Time derivative : Inport
  Constant11 : Constant  Value=278  VectorParams1D=off
  Integrator1 : Integrator
  Sum4 : Sum  Inputs=|++
  Out1 : Outport
  wires:
  Sum4/1 -> Out1/1
  Time derivative/1 -> Integrator1/1
  Integrator1/1 -> Sum4/2
  Constant11/1 -> Sum4/1

== system Backups/Input_Blowdown/n_a ==
  In1 : Inport
  Constant2 : Constant  Value=0.181
  Integrator2 : Integrator
  Sum2 : Sum  Inputs=|++
  O/P_Blowdown : Outport
  wires:
  In1/1 -> Integrator2/1
  Sum2/1 -> O/P_Blowdown/1
  Constant2/1 -> Sum2/1
  Integrator2/1 -> Sum2/2

== system Backups/Input_Blowdown/n_b ==
  In1 : Inport
  Constant : Constant  Value=0
  Integrator3 : Integrator
  Sum3 : Sum  Inputs=|++
  n_b : Outport
  wires:
  Sum3/1 -> n_b/1
  Constant/1 -> Sum3/1
  In1/1 -> Integrator3/1
  Integrator3/1 -> Sum3/2

== system Backups/Input_Blowdown1/A_injector ==
  Display1 : Display
  MATLAB Function1 : MATLAB Function  TreatAsAtomicUnit=on
  m_dot_des2 : Constant
  A_inj : Outport
  wires:
  MATLAB Function1/1(A_inj) -> A_inj/1, Display1/1
  m_dot_des2/1 -> MATLAB Function1/1(m_dot_des)

== system Backups/Input_Blowdown1/T ==
  Time derivative : Inport
  Constant11 : Constant  Value=278  VectorParams1D=off
  Integrator1 : Integrator
  Sum4 : Sum  Inputs=|++
  Out1 : Outport
  wires:
  Sum4/1 -> Out1/1
  Time derivative/1 -> Integrator1/1
  Integrator1/1 -> Sum4/2
  Constant11/1 -> Sum4/1

== system Backups/Input_Blowdown1/n_a ==
  In1 : Inport
  Constant2 : Constant  Value=0.181
  Integrator2 : Integrator
  Sum2 : Sum  Inputs=|++
  O/P_Blowdown : Outport
  wires:
  In1/1 -> Integrator2/1
  Sum2/1 -> O/P_Blowdown/1
  Constant2/1 -> Sum2/1
  Integrator2/1 -> Sum2/2

== system Backups/Input_Blowdown1/n_b ==
  In1 : Inport
  Constant : Constant  Value=0
  Integrator3 : Integrator
  Sum3 : Sum  Inputs=|++
  n_b : Outport
  wires:
  Sum3/1 -> n_b/1
  Constant/1 -> Sum3/1
  In1/1 -> Integrator3/1
  Integrator3/1 -> Sum3/2

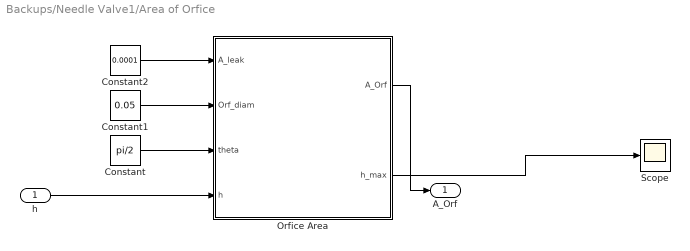
== system Backups/Needle Valve1/Area of Orfice ==
  h : Inport
  Constant : Constant  Value=pi/2
  Constant1 : Constant  Value=0.05
  Constant2 : Constant  Value=0.0001
  Orfice Area : MATLAB Function  TreatAsAtomicUnit=on
  Scope : Scope
  A_Orf : Outport
  wires:
  Constant1/1 -> Orfice Area/2(Orf_diam)
  Constant/1 -> Orfice Area/3(theta)
  h/1 -> Orfice Area/4(h)
  Orfice Area/1(A_Orf) -> A_Orf/1
  Constant2/1 -> Orfice Area/1(A_leak)
  Orfice Area/2(h_max) -> Scope/1

== system Backups/Needle Valve1/Height of Needle ==
  In1 : Inport
  Integrator : Integrator
  Sum : Sum  Inputs=|++
  h_init : Constant  Value=0.01
  h : Outport
  wires:
  In1/1 -> Integrator/1
  Sum/1 -> h/1  "h"
  Integrator/1 -> Sum/2
  h_init/1 -> Sum/1

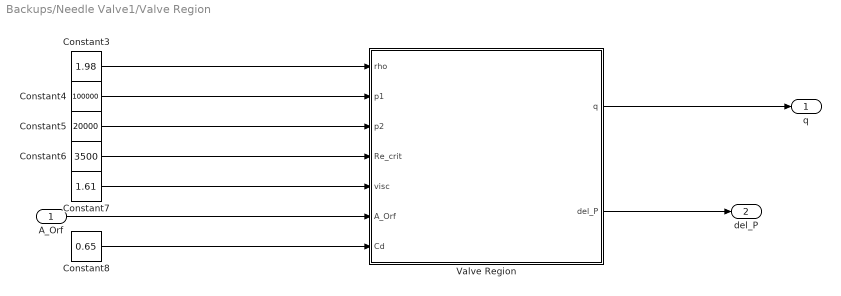
== system Backups/Needle Valve1/Valve Region ==
  A_Orf : Inport
  Constant3 : Constant  Value=1.98
  Constant4 : Constant  Value=100000
  Constant5 : Constant  Value=20000
  Constant6 : Constant  Value=3500
  Constant7 : Constant  Value=1.61
  Constant8 : Constant  Value=0.65
  Valve Region : MATLAB Function  TreatAsAtomicUnit=on
  q : Outport
  del_P : Outport  Port=2
  wires:
  Valve Region/2(del_P) -> del_P/1
  Constant7/1 -> Valve Region/5(visc)
  Constant4/1 -> Valve Region/2(p1)
  Constant8/1 -> Valve Region/7(Cd)
  A_Orf/1 -> Valve Region/6(A_Orf)
  Constant3/1 -> Valve Region/1(rho)
  Constant6/1 -> Valve Region/4(Re_crit)
  Valve Region/1(q) -> q/1
  Constant5/1 -> Valve Region/3(p2)

== matlab function Backups/Input_Needleboi/Cv ==
  data: Cv output; u input
function Cv = Cvcalc(u)
Cv = u/20;

% if (u<2)
%     Cv = u/20;
% % elseif(u>6&&u<9)
% % Cv=((1.1169*(u-5.95)^2))/100+0.03;
% else
%   Cv=0;
%     
% end
% 
%     
% % till 0.1
end

== matlab function Backups/MATLAB Function1 ==
  data: p2 input; p1 input; Cv input; sg input; Temp input; rho input; q output; MW input
function q   = Needleboi(p2,p1,Cv,sg,Temp,rho,MW)
%sg is specific gravity
p1_new=p1/98066.5;
p2_new=p2/98066.5;

del_p=p1_new-p2_new;
if (p2>0.5*p1)
    q=0.11362272*Cv*p1_new*(1-(2*del_p)/(3*p1_new))*sqrt((del_p/(p1_new*sg*Temp)))* rho/MW ...
       *101325/3.62e6 * 288/278 ;
    %L/min=6816 => *1.66667e-5
else
    q=0.471*0.11362272*Cv*p1_new*sqrt(1/(sg*Temp)) * rho/MW ...
       *101325/3.62e6* 288/278;
    %vol flow rate
end

== matlab function Backups/MATLAB Function4 ==
  data: dT output; dn_a output; dn_b output; m_dot output; n_a input; n_b input; T input; V input; A_inj input; m_tank input; Cd input; Pe input; P output; nPres input
function [dT, dn_a, dn_b, m_dot, P] = nox_blowdown(n_a, n_b, T, V, A_inj,m_tank,  Cd, Pe, nPres )
%OX_TANK_SIM Models thermochemical processes of blow-down in oxidizer tank.
%   Propellant Tank Pressurization Modeling for a Hybrid Rocket - Margaret
%   Mary Fernandez
%
%   INPUTS:
%       "n" = 1x2 vector of ox moles in tank (kmol).
%       "T" = ox tank temperature (K).
%       "V" = volume of ox tank (m^3).
%       "m_tank" = mass of oxidizer tank (kg).
%       "m_dot_prev" = ox mass flow rate of previous time step (kg/s).
%       "A_inj" = total orifice area of injector plate (m^2).
%       "Cd" = injector plate discharge coefficient.
%       "Pe" = pressure at exit of injector plate (Pa).
%
%   OUTPUTS:
%       "m_dot" = scalar ox mass flow rate (kg/s).
%       "dn" = 1x2 differential change in ox moles (kmol).
%       "dT" = differential change in ox tank temperature (K).
%       "P" = scalar internal pressure of ox tank (Pa).
%%%%%%%%%%%%%%%%%%%%%%%%%%%%%%%%%%%%%%%%%%%%%%%%%%%%%%%%%%%%%%%%%%%%%%%%%%%

%Perry's Chemical Engineers' Handbook Property Equations:
G1 = 96.512;           %Vapour pressure of N2O [Pa] coefficients
G2 = -4045;            % valid for Temp range [182.3 K - 309.57 K]
G3 = -12.277;
G4 = 2.886e-5;
G5 = 2;

Tc = 309.57;           % critical temperature of N2O [K]

J1 = 2.3215e7;         % heat of vaporization of N2O [J/kmol] coefficients
J2 = 0.384;            % valid for Temp range [182.3 K - 309.57 K]
J3 = 0;
J4 = 0;

% % heat capacity of N2 at constant pressure [J/(kmol*K)] coefficients
% % valid for Temp range [100 K - 1500 K]
% C1 = 0.28883e5; 
% C2 = 0;              
% C3 = 0;
% C4 = 0;
% C5 = 0;

D1 = 0.2934e5; % heat capacity of N2O gas at constant pressure [J/(kmol*K)] coefficients
D2 = 0.3236e5; % valid for Temp range [100 K - 1500 K]
D3 = 1.1238e3;
D4 = 0.2177e5;
D5 = 479.4; 

E1 = 6.7556e4; % heat capacity of N2O liquid at constant pressure [J/(kmol*K)] coefficients
E2 = 5.4373e1; % valid for Temp range [182.3 K - 200 K]
E3 = 0;
E4 = 0;
E5 = 0;
Q1 = 2.781;    % molar specific volume of liquid N2O [m^3/kmol] coefficients
Q2 = 0.27244;
Q3 = 309.57;
Q4 = 0.2882;

R  = 8314;      %Universal gas constant (J/kmol*K).
MW = 44.013;   %Molar mass of N2O (kg/kmol)​
% Calculate thermodynamic parameters as functions of temperature:
Vhat_l      = Q2^(1 + (1 - T/Q3)^Q4)/Q1;                    %Molar specific vol. of liq. N2O [m^3/kmol]
CVhat_g     = D1 + D2*((D3/T)/sinh(D3/T))^2 + ...
              D4*((D5/T)/cosh(D5/T))^2 - R;                 %Molar c_V of N2O gas [J/(kmol*K)]
CVhat_l     = E1 + E2*T + E3*T^2 + E4*T^3 + E5*T^4;         %Molar c_V of N2O liq.; approx. = c_P [J/(kmol*K)]
Tr          = T/Tc;                                         %Reduced temperature.
delta_Hv    = J1*(1 - Tr) ^ (J2 + J3*Tr + J4*Tr^2);         %Heat of vaporization of N2O [J/kmol]
P_sat       = exp(G1 + G2/T + G3*log(T) + G4*T^G5);         %Vapour P of N20 (Pa).
dP_sat      = (-G2/(T^2) + G3/T + G4*G5*T^(G5-1)) ...       %Derivative of vapour P with respect to T.
              * exp(G1 + G2/T + G3*log(T) + G4*T^G5);        
c_P         = (4.8 + 0.00322*T)*155.239;                    %Specific heat of tank, Aluminum [J/kg*K]

% 
%       P      = (nPres + n(2))*obj.utilities.R*T/(V - n(1)*Vhat_l);
%       a      = m_tank*c_P + nPres*CVhat_Pres + n(2)*CVhat_g + n(1)*CVhat_l;
%       RT     = P*Vhat_l;
%       e      = -delta_Hv + RT;
%       f      = -Cd*A_inj*sqrt(abs(2/MW*(P - Pe)/Vhat_l));
%       j      = -Vhat_l*P_sat;
%       k      = (V- n(1)*Vhat_l)*dP_sat;
%       l      = R*T;
%       q      = R*n(2);
%       Z      = (-f*(-j*a + (q - k)RT))/(a(l + j) + (q - k)*(e - RT));
%       W      = (-Z*(l*a + (q - k)*e))/(-j*a + (q - k)*RT);
%       dT     = (RT*W + e*Z)/a;


%Simplified expression definitions for solution:
P = (nPres+n_b)*R*T/(V - n_a*Vhat_l);
a = m_tank*c_P  + nPres*CVhat_l+n_b*CVhat_g + n_a*CVhat_l;
RT = P*Vhat_l;
e = -delta_Hv + R*T;
f = -Cd*A_inj*sqrt(abs(2/MW*(P - Pe)/Vhat_l));
j = -Vhat_l*P_sat;
k = (V - n_a*Vhat_l)*dP_sat;
l = R*T;
q = R*n_b;
Z = (-f*(-j*a + (q - k)*RT))/(a*(l + j) + (q - k)*(e - RT));
W = (-Z*(l*a + (q - k)*e))/(-j*a + (q - k)*RT);
%Time derivative of tank conditions
m_dot = -f*MW;          % Mass flow rate
dn_a    = W;    % Time derivative of nitrous amount
dn_b=Z;
dT    = (RT*W + e*Z)/a;  % Time derivative of tank temperature

end

== matlab function Backups/Input_Blowdown1/A_injector/MATLAB Function1 ==
  data: A_inj output; m_dot_des input
function A_inj  = A_inj(m_dot_des)
Cd=0.50;
MW=44;
P=3.62e6;
Pe=2.413e6;
Vhat_l=0.05;

A_inj=(m_dot_des)/(Cd*sqrt(abs(2/MW*(P - Pe)/Vhat_l))*MW);

== matlab function Backups/Input_Needleboi1/Cv ==
  data: Cv output; u input
function Cv = Cvcalc(u)
Cv = u/20;

% if (u<2)
%     Cv = u/20;
% % elseif(u>6&&u<9)
% % Cv=((1.1169*(u-5.95)^2))/100+0.03;
% else
%   Cv=0;
%     
% end
% 
%     
% % till 0.1
end

== matlab function Backups/MATLAB Function3 ==
  data: p2 input; p1 input; Cv input; sg input; Temp input; rho input; q output; MW input
function q   = Needleboi(p2,p1,Cv,sg,Temp,rho,MW)
%sg is specific gravity
p1_new=p1/98066.5;
p2_new=p2/98066.5;

del_p=p1_new-p2_new;
if (p2>0.5*p1)
    q=0.11362272*Cv*p1_new*(1-(2*del_p)/(3*p1_new))*sqrt((del_p/(p1_new*sg*Temp)))* rho/MW ...
       *101325/3.62e6 * 288/278 ;
    %L/min=6816 => *1.66667e-5
else
    q=0.471*0.11362272*Cv*p1_new*sqrt(1/(sg*Temp)) * rho/MW ...
       *101325/3.62e6* 288/278;
    %vol flow rate
end

== matlab function Backups/MATLAB Function5 ==
  data: dT output; dn_a output; dn_b output; m_dot output; n_a input; n_b input; T input; V input; A_inj input; m_tank input; Cd input; Pe input; P output; nPres input
function [dT, dn_a, dn_b, m_dot, P] = nox_blowdown(n_a, n_b, T, V, A_inj,m_tank,  Cd, Pe, nPres )
%OX_TANK_SIM Models thermochemical processes of blow-down in oxidizer tank.
%   Propellant Tank Pressurization Modeling for a Hybrid Rocket - Margaret
%   Mary Fernandez
%
%   INPUTS:
%       "n" = 1x2 vector of ox moles in tank (kmol).
%       "T" = ox tank temperature (K).
%       "V" = volume of ox tank (m^3).
%       "m_tank" = mass of oxidizer tank (kg).
%       "m_dot_prev" = ox mass flow rate of previous time step (kg/s).
%       "A_inj" = total orifice area of injector plate (m^2).
%       "Cd" = injector plate discharge coefficient.
%       "Pe" = pressure at exit of injector plate (Pa).
%
%   OUTPUTS:
%       "m_dot" = scalar ox mass flow rate (kg/s).
%       "dn" = 1x2 differential change in ox moles (kmol).
%       "dT" = differential change in ox tank temperature (K).
%       "P" = scalar internal pressure of ox tank (Pa).
%%%%%%%%%%%%%%%%%%%%%%%%%%%%%%%%%%%%%%%%%%%%%%%%%%%%%%%%%%%%%%%%%%%%%%%%%%%

%Perry's Chemical Engineers' Handbook Property Equations:
G1 = 96.512;           %Vapour pressure of N2O [Pa] coefficients
G2 = -4045;            % valid for Temp range [182.3 K - 309.57 K]
G3 = -12.277;
G4 = 2.886e-5;
G5 = 2;

Tc = 309.57;           % critical temperature of N2O [K]

J1 = 2.3215e7;         % heat of vaporization of N2O [J/kmol] coefficients
J2 = 0.384;            % valid for Temp range [182.3 K - 309.57 K]
J3 = 0;
J4 = 0;

% % heat capacity of N2 at constant pressure [J/(kmol*K)] coefficients
% % valid for Temp range [100 K - 1500 K]
% C1 = 0.28883e5; 
% C2 = 0;              
% C3 = 0;
% C4 = 0;
% C5 = 0;

D1 = 0.2934e5; % heat capacity of N2O gas at constant pressure [J/(kmol*K)] coefficients
D2 = 0.3236e5; % valid for Temp range [100 K - 1500 K]
D3 = 1.1238e3;
D4 = 0.2177e5;
D5 = 479.4; 

E1 = 6.7556e4; % heat capacity of N2O liquid at constant pressure [J/(kmol*K)] coefficients
E2 = 5.4373e1; % valid for Temp range [182.3 K - 200 K]
E3 = 0;
E4 = 0;
E5 = 0;
Q1 = 2.781;    % molar specific volume of liquid N2O [m^3/kmol] coefficients
Q2 = 0.27244;
Q3 = 309.57;
Q4 = 0.2882;

R  = 8314;      %Universal gas constant (J/kmol*K).
MW = 44.013;   %Molar mass of N2O (kg/kmol)​
% Calculate thermodynamic parameters as functions of temperature:
Vhat_l      = Q2^(1 + (1 - T/Q3)^Q4)/Q1;                    %Molar specific vol. of liq. N2O [m^3/kmol]
CVhat_g     = D1 + D2*((D3/T)/sinh(D3/T))^2 + ...
              D4*((D5/T)/cosh(D5/T))^2 - R;                 %Molar c_V of N2O gas [J/(kmol*K)]
CVhat_l     = E1 + E2*T + E3*T^2 + E4*T^3 + E5*T^4;         %Molar c_V of N2O liq.; approx. = c_P [J/(kmol*K)]
Tr          = T/Tc;                                         %Reduced temperature.
delta_Hv    = J1*(1 - Tr) ^ (J2 + J3*Tr + J4*Tr^2);         %Heat of vaporization of N2O [J/kmol]
P_sat       = exp(G1 + G2/T + G3*log(T) + G4*T^G5);         %Vapour P of N20 (Pa).
dP_sat      = (-G2/(T^2) + G3/T + G4*G5*T^(G5-1)) ...       %Derivative of vapour P with respect to T.
              * exp(G1 + G2/T + G3*log(T) + G4*T^G5);        
c_P         = (4.8 + 0.00322*T)*155.239;                    %Specific heat of tank, Aluminum [J/kg*K]

% 
%       P      = (nPres + n(2))*obj.utilities.R*T/(V - n(1)*Vhat_l);
%       a      = m_tank*c_P + nPres*CVhat_Pres + n(2)*CVhat_g + n(1)*CVhat_l;
%       RT     = P*Vhat_l;
%       e      = -delta_Hv + RT;
%       f      = -Cd*A_inj*sqrt(abs(2/MW*(P - Pe)/Vhat_l));
%       j      = -Vhat_l*P_sat;
%       k      = (V- n(1)*Vhat_l)*dP_sat;
%       l      = R*T;
%       q      = R*n(2);
%       Z      = (-f*(-j*a + (q - k)RT))/(a(l + j) + (q - k)*(e - RT));
%       W      = (-Z*(l*a + (q - k)*e))/(-j*a + (q - k)*RT);
%       dT     = (RT*W + e*Z)/a;


%Simplified expression definitions for solution:
P = (nPres+n_b)*R*T/(V - n_a*Vhat_l);
a = m_tank*c_P  + nPres*CVhat_l+n_b*CVhat_g + n_a*CVhat_l;
RT = P*Vhat_l;
e = -delta_Hv + R*T;
f = -Cd*A_inj*sqrt(abs(2/MW*(P - Pe)/Vhat_l));
j = -Vhat_l*P_sat;
k = (V - n_a*Vhat_l)*dP_sat;
l = R*T;
q = R*n_b;
Z = (-f*(-j*a + (q - k)*RT))/(a*(l + j) + (q - k)*(e - RT));
W = (-Z*(l*a + (q - k)*e))/(-j*a + (q - k)*RT);
%Time derivative of tank conditions
m_dot = -f*MW;          % Mass flow rate
dn_a    = W;    % Time derivative of nitrous amount
dn_b=Z;
dT    = (RT*W + e*Z)/a;  % Time derivative of tank temperature

end

== matlab function Backups/Cv/Cv ==
  data: Cv output; u input
function Cv = Cvcalc(u)
Cv = u/20;

% if (u<2)
%     Cv = u/20;
% % elseif(u>6&&u<9)
% % Cv=((1.1169*(u-5.95)^2))/100+0.03;
% else
%   Cv=0;
%     
% end
% 
%     
% % till 0.1
end

== matlab function Backups/MATLAB Function6 ==
  data: Cv input; p2 input; sg input; MW input; Temp input; p1 input; q output; mdot output; Z input
function [q, mdot]   = Needle_valve(Cv,p2,sg,MW,Temp,p1,Z)
    %sg is specific gravity
    
    p1_new=p1/98066.5;
    p2_new=p2/98066.5;

    del_p=p1_new-p2_new;
    
    R = 8314 / 28;
    rho = p1 / (R * Z * Temp);

    if (p2>0.5*p1)
        q=0.11362272*Cv*p1_new*(1-(2*del_p)/(3*p1_new))*sqrt((del_p/(p1_new*sg*Temp)))* rho/MW * (101325/p1 * Temp/288);
        mdot=q*MW;
    else
        q=0.471*0.11362272*Cv*p1_new*sqrt(1/(sg*Temp)) * rho/MW * (101325/p1 * Temp/288);
        mdot=q*MW;
    end

end

== matlab function Backups/MATLAB Function7 ==
  data: P input; A_inj output; m_dot_des input; Cd input; Pe input
function A_inj  = A_inj(P, m_dot_des, Cd, Pe)
MW=44;
Vhat_l=0.05;

A_inj=(m_dot_des)/(Cd*sqrt(abs(2/MW*(P - Pe)/Vhat_l))*MW);
